simulink model "example3"  (R2019b)
settings: Solver=VariableStepAuto  StartTime=0.0  StopTime=10.0  RelTol=1e-3
settings Model: Creator=davis  LastModifiedBy=davis

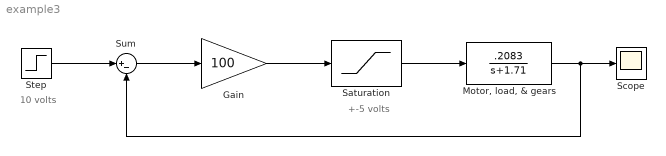
== system example3 ==
  note: +-5 volts
  note: 10 volts
  Gain : Gain  Gain=100
  "Motor, load, & gears" : TransferFcn  Numerator=[.2083]  Denominator=[1 1.71]
  Saturation : Saturate  UpperLimit=5  LowerLimit=-5
  Scope : Scope
  Step : Step  Time=0  After=10  SampleTime=0
  Sum : Sum  Inputs=|+-
  wires:
  Step/1 -> Sum/1
  Sum/1 -> Gain/1
  Gain/1 -> Saturation/1
  Saturation/1 -> "Motor, load, & gears"/1
  "Motor, load, & gears"/1 -> Sum/2, Scope/1
